simulink model "ref_subsystem_test"  (Simulink 8.7)
settings: Solver=FixedStepAuto  StartTime=0.0  StopTime=10.0  RelTol=1e-3
settings Model: Creator=arnaud  LastModifiedBy=hamza
settings DataIOCC: SaveFormat=Structure  SaveOutput=off  SaveTime=off
settings DebuggingCC: UnderspecifiedInitializationDetection=Simplified  MergeDetectMultiDrivingBlocksExec=error  SolverPrmCheckMsg=warning
settings ConfigComp: CovSFcnEnable=off

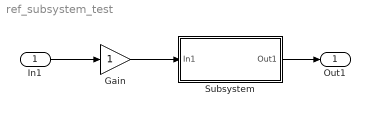
== system ref_subsystem_test ==
  In1 : Inport  OutDataTypeStr=double  PortDimensions=1  SampleTime=0
  Gain : Gain
  Subsystem : Subsystem  TreatAsAtomicUnit=on
  Out1 : Outport  OutDataTypeStr=double  PortDimensions=1  SampleTime=0
  wires:
  In1/1 -> Gain/1
  Subsystem/1(Out1) -> Out1/1
  Gain/1 -> Subsystem/1(In1)

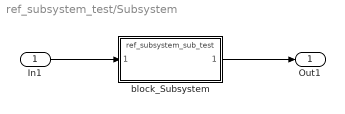
== system ref_subsystem_test/Subsystem ==
  In1 : Inport
  block_Subsystem : ModelReference  ModelNameDialog=ref_subsystem_sub_test.mdl  SimulationMode=Normal  ModelReferenceVersion=1.12
  Out1 : Outport
  wires:
  In1/1 -> block_Subsystem/1
  block_Subsystem/1 -> Out1/1
